simulink model "DeadZonePWM01"  (R2021b)
settings: Solver=ode23tb  StartTime=0.0  StopTime=30.0  MaxStep=1.0e-5  MinStep=1.0e-12  RelTol=1e-3
values from neighbouring files (symbols this model uses):
  kpot = 1.0    (= 1)    [ini_sim.m]
  kuadj = umax/(umax-DZmax)    (= 1.07296137339)    [ini_sim.m]
  N = 9.0    (= 9)    [ini_sim.m]
  taum = 0.3    [ini_sim.m]
  Tsw = 1/Fsw    [ini_sim.m]
  umax = 5.0    (= 5)    [ini_sim.m]
  umin = -umax    (= -5)    [ini_sim.m]
  Vm = 5.0    (= 5)    [ini_sim.m]
undefined symbols (not defined in the file or in its folder): kc, km
libraries: simulink x1
settings Model: Creator=rgrino  LastModifiedBy=rgrino
settings SolverCC: InitialStep=1.0e-8

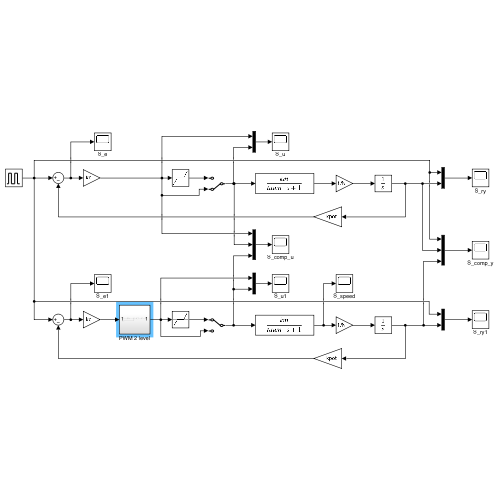
[thumbnail: Simulink's stored preview of the top-level diagram]
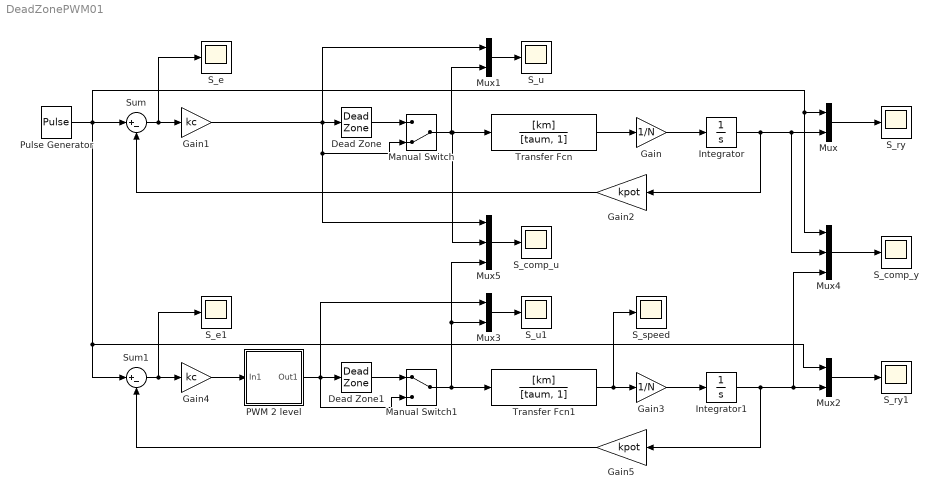
== system DeadZonePWM01 ==
  Dead Zone : DeadZone  LowerValue=DZmin  UpperValue=DZmax  SaturateOnIntegerOverflow=on
  Dead Zone1 : DeadZone  LowerValue=DZmin  UpperValue=DZmax  SaturateOnIntegerOverflow=on
  Gain : Gain  Gain=1/N
  Gain1 : Gain  Gain=kc
  Gain2 : Gain  Gain=kpot
  Gain3 : Gain  Gain=1/N
  Gain4 : Gain  Gain=kc
  Gain5 : Gain  Gain=kpot
  Integrator : Integrator
  Integrator1 : Integrator
  Manual Switch : ManualSwitch  CurrentSetting=0
  Manual Switch1 : ManualSwitch
  Mux{,1..3} (4 alike) : Mux  Inputs=2
  Mux4 : Mux  Inputs=3
  Mux5 : Mux  Inputs=3
  PWM 2 level : Subsystem
  Pulse Generator : DiscretePulseGenerator  PulseType=Time based  Amplitude=2  Period=10  PulseWidth=50
  S_comp_u : Scope
  S_comp_y : Scope
  S_e : Scope
  S_e1 : Scope
  S_ry : Scope
  S_ry1 : Scope
  S_speed : Scope
  S_u : Scope
  S_u1 : Scope
  Sum : Sum  Inputs=|+-
  Sum1 : Sum  Inputs=|+-
  Transfer Fcn : TransferFcn  Numerator=[km]  Denominator=[taum, 1]
  Transfer Fcn1 : TransferFcn  Numerator=[km]  Denominator=[taum, 1]
  wires:
  Gain/1 -> Integrator/1
  Transfer Fcn/1 -> Gain/1
  Gain1/1 -> Mux1/1, Mux5/1, Manual Switch/2, Dead Zone/1
  Sum/1 -> S_e/1, Gain1/1
  Integrator/1 -> Gain2/1, Mux4/2, Mux/2
  Pulse Generator/1 -> Sum1/1, Mux2/1, Mux4/1, Mux/1, Sum/1
  Mux/1 -> S_ry/1
  Gain2/1 -> Sum/2
  Manual Switch/1 -> Mux1/2, Mux5/2, Transfer Fcn/1
  Dead Zone/1 -> Manual Switch/1
  Mux1/1 -> S_u/1
  Gain3/1 -> Integrator1/1
  Transfer Fcn1/1 -> S_speed/1, Gain3/1
  Gain5/1 -> Sum1/2
  Manual Switch1/1 -> Mux5/3, Mux3/2, Transfer Fcn1/1
  Mux2/1 -> S_ry1/1
  Sum1/1 -> S_e1/1, Gain4/1
  Integrator1/1 -> Gain5/1, Mux4/3, Mux2/2
  Dead Zone1/1 -> Manual Switch1/1
  Mux3/1 -> S_u1/1
  PWM 2 level/1(Out1) -> Mux3/1, Manual Switch1/2, Dead Zone1/1
  Mux4/1 -> S_comp_y/1
  Mux5/1 -> S_comp_u/1
  Gain4/1 -> PWM 2 level/1(In1)

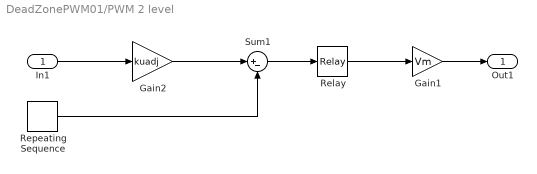
== system DeadZonePWM01/PWM 2 level ==
  In1 : Inport
  Gain1 : Gain  Gain=Vm
  Gain2 : Gain  Gain=kuadj
  Relay : Relay  OffSwitchValue=-eps  OffOutputValue=-1
  Repeating Sequence : simulink/Sources/Repeating Sequence  rep_seq_t=[0, Tsw/2, Tsw]  rep_seq_y=[umax, umin, umax]
  Sum1 : Sum  Inputs=|+-
  Out1 : Outport
  wires:
  Repeating Sequence/1 -> Sum1/2
  Sum1/1 -> Relay/1
  Relay/1 -> Gain1/1
  Gain1/1 -> Out1/1
  Gain2/1 -> Sum1/1
  In1/1 -> Gain2/1
